simulink model "LotkaVolterra"  (R2018b)
settings: Solver=VariableStepAuto  StartTime=0.0  StopTime=100  RelTol=1e-3
values from neighbouring files (symbols this model uses):
  K_1 = 4    [main.m]
  k_1 = 1    [main.m]
  K_2 = 18    [main.m]
  k_2 = 1    [main.m]
  k_3 = 1    [main.m]
  k_4 = 1    [main.m]
  K_d = 7    [main.m]
  K_p = 5    [main.m]
undefined symbols (not defined in the file or in its folder): sigbuilder_block
settings Model: Creator=Kakedral  LastModifiedBy=Kakedral

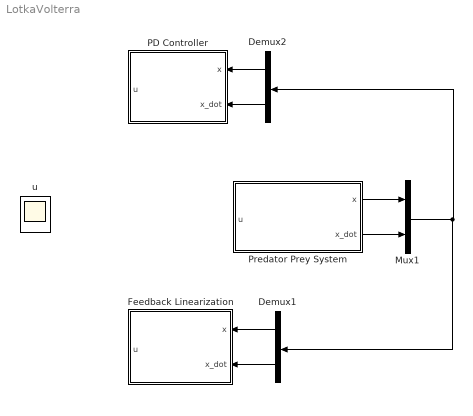
== system LotkaVolterra ==
  Demux1 : Demux  Outputs=2
  Demux2 : Demux  Outputs=2
  Feedback Linearization : Subsystem
  Mux1 : Mux  Inputs=2
  PD Controller : Subsystem
  "Predator Prey System " : Subsystem
  u : Scope
  wires:
  "Predator Prey System "/2(x_dot) -> Mux1/2
  Mux1/1 -> Demux1/1, Demux2/1
  "Predator Prey System "/1(x) -> Mux1/1
  Demux2/1 -> PD Controller/1("x ")
  Demux2/2 -> PD Controller/2(x_dot)
  Demux1/1 -> Feedback Linearization/1(x)
  Demux1/2 -> Feedback Linearization/2(x_dot)

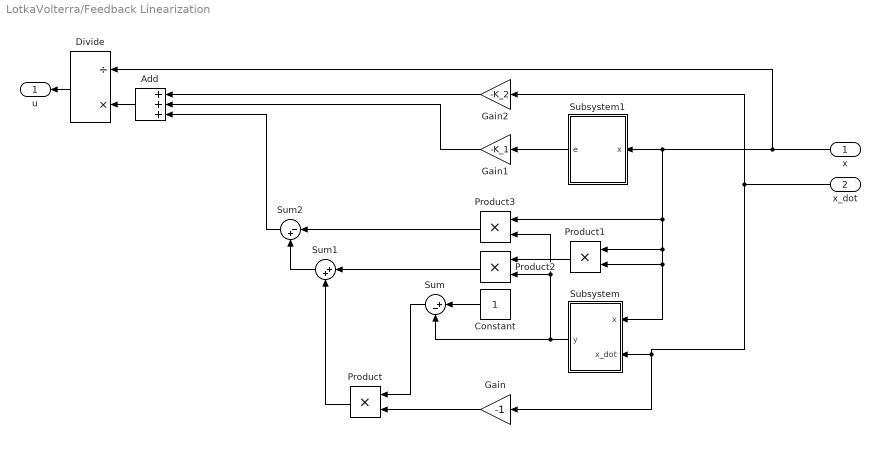
== system LotkaVolterra/Feedback Linearization ==
  x : Inport
  x_dot : Inport  Port=2
  Add : Sum  Inputs=+++
  Constant : Constant
  Divide : Product  Inputs=/*
  Gain : Gain  Gain=-1
  Gain1 : Gain  Gain=-K_1
  Gain2 : Gain  Gain=-K_2
  Product{,1..3} (4 alike) : Product
  Subsystem : Subsystem
  Subsystem1 : Subsystem
  Sum : Sum  Inputs=|+-
  Sum1 : Sum  Inputs=|++
  Sum2 : Sum  Inputs=|-+
  u : Outport
  wires:
  Product2/1 -> Sum1/1
  x/1 -> Divide/1, Product3/1, Product1/1, Subsystem/1(x), Product1/2, Subsystem1/1(x)
  Constant/1 -> Sum/1
  Sum/1 -> Product/1
  Subsystem/1(y) -> Product2/2, Product3/2, Sum/2
  Product/1 -> Sum1/2
  Divide/1 -> u/1
  Product3/1 -> Sum2/1
  Product1/1 -> Product2/1
  Sum1/1 -> Sum2/2
  Subsystem1/1(e) -> Gain1/1
  x_dot/1 -> Gain2/1, Gain/1, Subsystem/2(x_dot)
  Gain1/1 -> Add/2
  Sum2/1 -> Add/3
  Gain/1 -> Product/2
  Gain2/1 -> Add/1
  Add/1 -> Divide/2

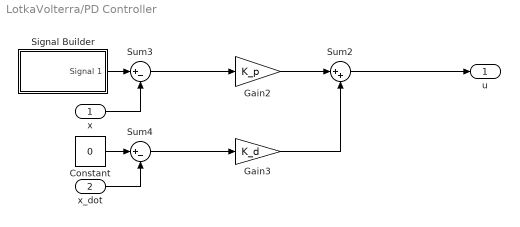
== system LotkaVolterra/PD Controller ==
  "x " : Inport
  x_dot : Inport  Port=2
  Constant : Constant  Value=0  VectorParams1D=off
  Gain2 : Gain  Gain=K_p
  Gain3 : Gain  Gain=K_d
  Signal Builder : Subsystem  Tag=STV Subsys  LoadFcn=sigbuilder_block('load');  StartFcn=sigbuilder_block('start');  StopFcn=sigbuilder_block('stop');  ClipboardFcn=sigbuilder_block('clipboard');  mask(Sigbuilder block){tuvar=[0:10]}
      mask help: Simulink:masks:SigbuilderBlock_MD
      mask init:
      | if ~strcmp(get_param(bdroot(gcbh),'SimulationStatus'),'stopped') tuvar = sigbuilder_block('maskInit'); end
      settings: CopyFcn=sigbuilder_block('copy');  DeleteFcn=sigbuilder_block('delete');  ModelCloseFcn=sigbuilder_block('modelClose');  PreSaveFcn=sigbuilder_block('preSave');  PauseFcn=sigbuilder_block('pause');  ContinueFcn=sigbuilder_block('continue');  NameChangeFcn=sigbuilder_block('namechange');  OpenFcn=sigbuilder_block('open',[437.6 199.2 550.4 400 ]);  CloseFcn=sigbuilder_block('close');
      mask Display: plot(0, 0, 100, 100,[2, 2, 32, 32, 2], [68, 8, 8, 68, 68],[32, 2], [38, 38], [32, 19, 2],[53, 60, 44], [32, 17, 17, 2],[16, 16, 31, 31]);txt = getActiveGroup(gcbh);text(2, 100, txt,'verticalAlignment', 'top');
  Sum2 : Sum  Inputs=|++
  Sum3 : Sum  Inputs=|+-
  Sum4 : Sum  Inputs=|+-
  "u " : Outport
  wires:
  Constant/1 -> Sum4/1
  "x "/1 -> Sum3/2
  Gain3/1 -> Sum2/2
  x_dot/1 -> Sum4/2
  Sum2/1 -> "u "/1
  Signal Builder/1(Signal 1) -> Sum3/1
  Sum3/1 -> Gain2/1
  Sum4/1 -> Gain3/1
  Gain2/1 -> Sum2/1

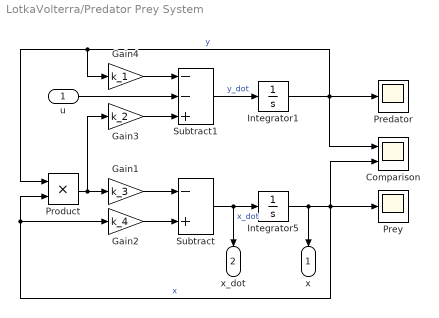
== system LotkaVolterra/Predator Prey System  ==
  "u " : Inport
  "Comparison " : Scope  NumInputPorts=2
  Gain1 : Gain  Gain=k_3
  Gain2 : Gain  Gain=k_4
  Gain3 : Gain  Gain=k_2
  Gain4 : Gain  Gain=k_1
  Integrator1 : Integrator  InitialCondition=4
  Integrator5 : Integrator  InitialCondition=6
  Predator : Scope
  Prey : Scope
  Product : Product
  Subtract : Sum  Inputs=-+
  Subtract1 : Sum  Inputs=--+
  x : Outport
  x_dot : Outport  Port=2
  wires:
  Integrator1/1 -> "Comparison "/1, Product/1, Gain4/1, Predator/1  "y"
  Gain4/1 -> Subtract1/1
  Product/1 -> Gain1/1, Gain3/1
  Subtract/1 -> Integrator5/1, x_dot/1  "x_dot"
  Integrator5/1 -> x/1, Gain2/1, Product/2, "Comparison "/2, Prey/1  "x"
  Gain1/1 -> Subtract/1
  Gain2/1 -> Subtract/2
  Subtract1/1 -> Integrator1/1  "y_dot"
  Gain3/1 -> Subtract1/3
  "u "/1 -> Subtract1/2

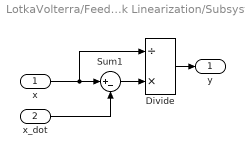
== system LotkaVolterra/Feedback Linearization/Subsystem ==
  x : Inport
  x_dot : Inport  Port=2
  Divide : Product  Inputs=/*
  Sum1 : Sum  Inputs=|+-
  y : Outport
  wires:
  x/1 -> Divide/1, Sum1/1
  Sum1/1 -> Divide/2
  Divide/1 -> y/1
  x_dot/1 -> Sum1/2

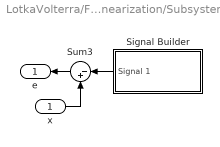
== system LotkaVolterra/Feedback Linearization/Subsystem1 ==
  x : Inport
  Signal Builder : Subsystem  Tag=STV Subsys  LoadFcn=sigbuilder_block('load');  StartFcn=sigbuilder_block('start');  StopFcn=sigbuilder_block('stop');  ClipboardFcn=sigbuilder_block('clipboard');  mask(Sigbuilder block){tuvar=[0:10]}
      mask help: Simulink:masks:SigbuilderBlock_MD
      mask init:
      | if ~strcmp(get_param(bdroot(gcbh),'SimulationStatus'),'stopped') tuvar = sigbuilder_block('maskInit'); end
      settings: CopyFcn=sigbuilder_block('copy');  DeleteFcn=sigbuilder_block('delete');  ModelCloseFcn=sigbuilder_block('modelClose');  PreSaveFcn=sigbuilder_block('preSave');  PauseFcn=sigbuilder_block('pause');  ContinueFcn=sigbuilder_block('continue');  NameChangeFcn=sigbuilder_block('namechange');  OpenFcn=sigbuilder_block('open',[437.6 199.2 550.4 400 ]);  CloseFcn=sigbuilder_block('close');
      mask Display: plot(0, 0, 100, 100,[2, 2, 32, 32, 2], [68, 8, 8, 68, 68],[32, 2], [38, 38], [32, 19, 2],[53, 60, 44], [32, 17, 17, 2],[16, 16, 31, 31]);txt = getActiveGroup(gcbh);text(2, 100, txt,'verticalAlignment', 'top');
  Sum3 : Sum  Inputs=|-+
  e : Outport
  wires:
  x/1 -> Sum3/2
  Sum3/1 -> e/1
  Signal Builder/1(Signal 1) -> Sum3/1

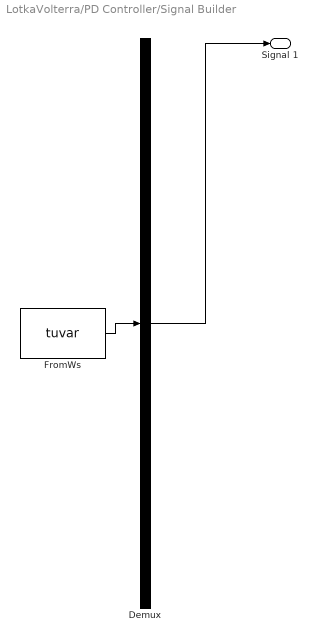
== system LotkaVolterra/PD Controller/Signal Builder ==
  Demux : Demux  Tag=STV Demux  Outputs=1
  FromWs : FromWorkspace  Tag=STV FromWs  VariableName=tuvar  SampleTime=0
      SigBuilderData=|
      | common.afterFinalStr = 'Extrapolate'
      | common.sampleTime = 0
      | dataSet.timeRange = [0 50]
      | dataSet.name = 'Group 1'
      | sbobj.Groups.Name = 'Group 1'
      | sbobj.Groups.Signals.Name = 'Signal 1'
      | sbobj.Groups.Signals.XData = [0 7.5 7.5 50]
      | sbobj.Groups.Signals.YData = [5 5 7.02 7.02]
      | sbobj.Groups.TimeRange = [0 50]
  Signal 1 : Outport  Tag=STV Outport
  wires:
  Demux/1 -> Signal 1/1
  FromWs/1 -> Demux/1

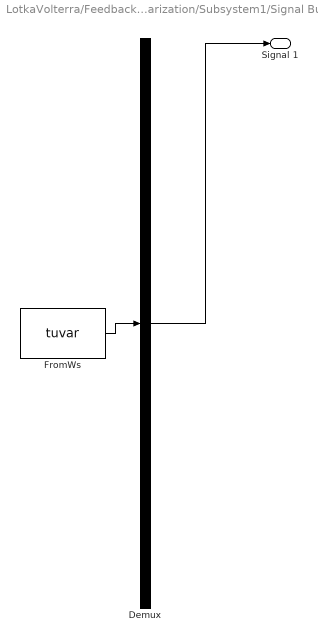
== system LotkaVolterra/Feedback Linearization/Subsystem1/Signal Builder ==
  Demux : Demux  Tag=STV Demux  Outputs=1
  FromWs : FromWorkspace  Tag=STV FromWs  VariableName=tuvar  SampleTime=0
      SigBuilderData=|
      | common.afterFinalStr = 'Extrapolate'
      | common.sampleTime = 0
      | dataSet.timeRange = [0 50]
      | dataSet.name = 'Group 1'
      | sbobj.Groups.Name = 'Group 1'
      | sbobj.Groups.Signals.Name = 'Signal 1'
      | sbobj.Groups.Signals.XData = [0 7.5 7.5 50]
      | sbobj.Groups.Signals.YData = [5 5 7.02 7.02]
      | sbobj.Groups.TimeRange = [0 50]
  Signal 1 : Outport  Tag=STV Outport
  wires:
  Demux/1 -> Signal 1/1
  FromWs/1 -> Demux/1
